simulink model "Model_1"  (R2020b)
settings: Solver=VariableStepAuto  StartTime=0.0  StopTime=10.0  RelTol=1e-3
values from neighbouring files (symbols this model uses):
  b = 0.1    [S1.m]
  J = 0.01    [S1.m]
  K = 0.01    [S1.m]
  L = 0.5    [S1.m]
  R = 1    [S1.m]
settings Model: Creator=Diwakar Reddy  LastModifiedBy=Diwakar Reddy

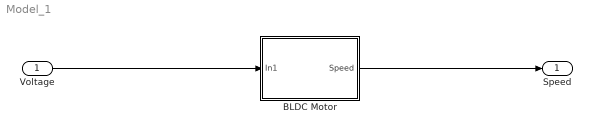
== system Model_1 ==
  Voltage : Inport
  BLDC Motor : Subsystem
  Speed : Outport
  wires:
  Voltage/1 -> BLDC Motor/1(In1)
  BLDC Motor/1(Speed) -> Speed/1

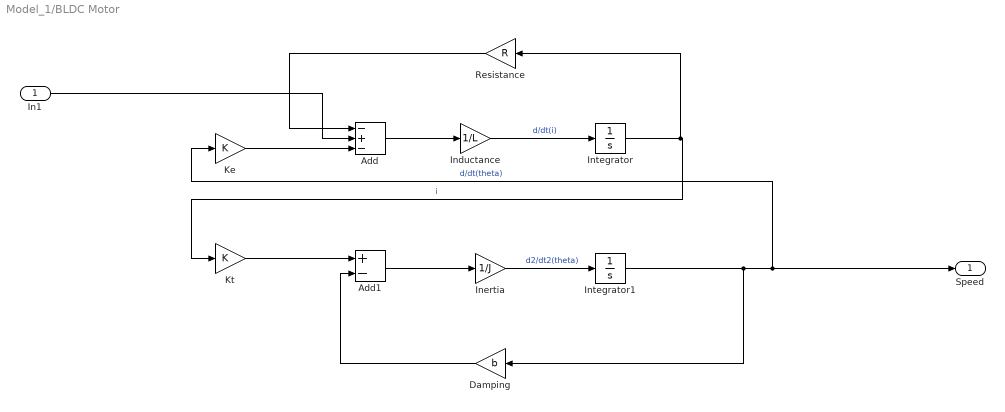
== system Model_1/BLDC Motor ==
  In1 : Inport
  Add : Sum  Inputs=-+-
  Add1 : Sum  Inputs=+-
  Damping : Gain  Gain=b
  Inductance : Gain  Gain=1/L
  Inertia : Gain  Gain=1/J
  Integrator : Integrator
  Integrator1 : Integrator
  Ke : Gain  Gain=K
  Kt : Gain  Gain=K
  Resistance : Gain  Gain=R
  Speed : Outport
  wires:
  Kt/1 -> Add1/1
  Inductance/1 -> Integrator/1  "d/dt(i)"
  Resistance/1 -> Add/1
  Integrator/1 -> Resistance/1, Kt/1  "i"
  Ke/1 -> Add/3
  Add/1 -> Inductance/1
  Integrator1/1 -> Speed/1, Ke/1, Damping/1  "d/dt(theta)"
  Inertia/1 -> Integrator1/1  "d2/dt2(theta)"
  Damping/1 -> Add1/2
  Add1/1 -> Inertia/1
  In1/1 -> Add/2
